simulink model "soc_dvbs2_fpga"  (R2025b)
settings: Solver=FixedStepDiscrete  StartTime=0.0  StopTime=0  RelTol=1e-3
InitFcn:
  | soc_dvbs2_init;
values from neighbouring files (symbols this model uses):
  Rsym = 4e6    (= 4000000)    [soc_dvbs2_init.m]
  soc_dvbs2_txPacketBits = [1 1 0 1 0 1 1 1 0 1 1 1 ... (2972 elements, 2972x1)]    [soc_dvbs2_txPacketBits.mat]
  syncWord = (dec2bin(hex2dec('AC')) - '0').'    [soc_dvbs2_init.m]
  txDataOut = txobj(frameBits(:))    [soc_dvbs2_init.m]
  txFiltCoeff = txobj.pTxFilterCoeff    [soc_dvbs2_init.m]
undefined symbols (not defined in the file or in its folder): Add, coefficientsLog, coefficientsSqrt1, coefficientsSqrt2, dataBits, designMultirateFIR, noisePow, NumBits1, NumBits2, seedsURNG1, seedsURNG2, Shift, Slope1, Slope2, soc_dvbs2_designFIRFilter, txDataOutS1, txDataOutS10, txDataOutS12, txDataOutS13, txDataOutS14, txDataOutS15, txDataOutS16, txDataOutS18, txDataOutS19, txDataOutS2, txDataOutS20, txDataOutS21, txDataOutS22, txDataOutS24, txDataOutS25, txDataOutS26, txDataOutS27, txDataOutS3, txDataOutS4, txDataOutS5, txDataOutS6, txDataOutS7, txDataOutS8, txDataOutS9
libraries: simulink x214, hdlsllib x211, dspsigops x22, dsphdlfiltering2 x8, dsphdlsigops2 x5, commseqgen3 x5, dsphdlmathfun2 x3, hwlogicconnlib x2, whdledac x2, commhdlcrc x2, whdlutilities x1, whdlmod x1
(part 12 of 12)

== matlab function soc_dvbs2_fpga/DVBS2/DVBS2 TxRx/DVB-S2 HDL Receiver/Demod Deinterleave and FECDecode/DVBS2 HDL Deinterleaver/RAM Address Generator/Read Offset Address/Read Offset Address Signals Generator ==
  data: maxR input; chkwrAddrEnd input; maxC input; modcodIs12 input; wrAddr input; curCorROut output; maxRorCOut output; curRorCOut output; modcodIs12Out output; startOut output; endOut output; wrEnb input; readValid output; isInterleave parameter
function [curCorROut,maxRorCOut,curRorCOut,modcodIs12Out,startOut,endOut,readValid] = readAddrCtrl(maxR,chkwrAddrEnd,maxC,modcodIs12,wrAddr,wrEnb,isInterleave)
%#codegen

    persistent rdEnb rdEnbOld startOutReg;
    persistent curR curC vMaxR vMaxC wrIdx rdIdx;
    persistent framCnt vModCodIs12;
    persistent curCorROutReg maxRorCOutReg curRorCOutReg modcodIs12OutReg;

    if isempty(rdEnb)
        rdEnb           = false;
%         rdEnbPrev       = false;
        rdEnbOld        = false;
        curR            = cast(0,'like',maxR);
        curC            = cast(0,'like',maxC);
        wrIdx           = fi(0,0,3,0,hdlfimath);
        rdIdx           = fi(0,0,3,0,hdlfimath);
        vMaxR           = cast(zeros(8,1),'like',maxR);
        vMaxC           = cast(zeros(8,1),'like',maxC);
        vModCodIs12     = false(8,1);
        startOutReg     = false;
        framCnt         = fi(0,0,3,0,hdlfimath);
        
        % XorY => Store X for Interleaver and Y for Deinterleaver
        if isInterleave        
            curCorROutReg   = curC;
            maxRorCOutReg   = vMaxR(1);
            curRorCOutReg   = curR;
        else
            curCorROutReg   = curR;
            maxRorCOutReg   = vMaxC(1);
            curRorCOutReg   = curC;
        end
        
        modcodIs12OutReg = vModCodIs12(1);
    end
    
    curCorROut   = curCorROutReg;
    maxRorCOut   = maxRorCOutReg;
    curRorCOut   = curRorCOutReg;
    modcodIs12Out = modcodIs12OutReg;
    readValid = rdEnbOld;
    startOut  = startOutReg; 
    
    endOut = false;
    if rdEnbOld
        if (isInterleave && (curC == (vMaxC(rdIdx+1)-1))) || (~isInterleave && (curR == (vMaxR(rdIdx+1)-1)))
            if isInterleave
                curC(:) = 0;
            else
                curR(:) = 0;
            end 
            if (~isInterleave && (curC == (vMaxC(rdIdx+1)-1))) || (isInterleave && (curR == (vMaxR(rdIdx+1)-1)))
                if ~isInterleave
                    curC(:) = 0;
                else
                    curR(:) = 0;
                end
                framCnt(:) = framCnt - 1;
                if framCnt == 0
                    rdEnb(:) = false;
                end
                endOut = true;
                if rdIdx == 7
                    rdIdx(:) = 0;
                else
                    rdIdx(:) = rdIdx + 1;
                end
            else
                if isInterleave
                    curR(:) = curR + 1;
                else
                    curC(:) = curC + 1;
                end
            end
        else
            if isInterleave
                curC(:) = curC + 1;
            else
                curR(:) = curR + 1;
            end
        end
    end
    
    if vModCodIs12(rdIdx+1) && curC == 0
        curCAdj = cast(2,'like',curC);
    elseif vModCodIs12(rdIdx+1) && curC == 2
        curCAdj = cast(0,'like',curC);
    else
        curCAdj = curC;
    end
    
    
    if isInterleave
        curCorROutReg    = curCAdj;
        maxRorCOutReg    = vMaxR(rdIdx+1);
        curRorCOutReg    = curR;
    else
        curCorROutReg    = curR;
        maxRorCOutReg    = vMaxC(rdIdx+1);
        curRorCOutReg    = curCAdj;
    end
    
    modcodIs12OutReg = vModCodIs12(rdIdx+1);

    startOutReg = rdEnb && (curR==0) && (curC==0);
    rdEnbOld = rdEnb;
%     rdEnbPrev = wrEnb && (wrAddr == chkwrAddrEnd);
    
    if wrEnb && (wrAddr == chkwrAddrEnd)
        framCnt(:) = framCnt + 1;
        rdEnb(:) = true;
        vModCodIs12(wrIdx+1) = modcodIs12;
        vMaxR(wrIdx+1) = maxR;
        vMaxC(wrIdx+1) = maxC;
        if wrIdx == 7
            wrIdx(:) = 0;
        else
            wrIdx(:) = wrIdx + 1;
        end
    end
    
end

== matlab function soc_dvbs2_fpga/DVBS2/DVBS2 TxRx/Channel/AWGN Generator/Unit Variance Gaussian Noise/logImplementation/log/RangeReduction/leadingZeroDetector ==
  data: x input; exp_e output
function exp_e=leadingZeroDetector(x)
temp = 0;
flag=1.0e+14 *[0.000000000000020
   0.000000000000040
   0.000000000000080
   0.000000000000160
   0.000000000000320
   0.000000000000640
   0.000000000001280
   0.000000000002560
   0.000000000005120
   0.000000000010240
   0.000000000020480
   0.000000000040960
   0.000000000081920
   0.000000000163840
   0.000000000327680
   0.000000000655360
   0.000000001310720
   0.000000002621440
   0.000000005242880
   0.000000010485760
   0.000000020971520
   0.000000041943040
   0.000000083886080
   0.000000167772160
   0.000000335544320
   0.000000671088640
   0.000001342177280
   0.000002684354560
   0.000005368709120
   0.000010737418240
   0.000021474836480
   0.000042949672960
   0.000085899345920
   0.000171798691840
   0.000343597383680
   0.000687194767360
   0.001374389534720
   0.002748779069440
   0.005497558138880
   0.010995116277760
   0.021990232555520
   0.043980465111040
   0.087960930222080
   0.175921860444160
   0.351843720888320
   0.703687441776640
   1.407374883553280
   2.814749767106560];

% else
%     while( )
%         temp = temp+1;
%         flag()=flag()*2;
%     end
% end
% 
% end
if(x == 0)
     temp = 49;
elseif (x*flag(1)>1)
        temp=1;
elseif (x*flag(2)>1)
        temp=2;
elseif (x*flag(3)>1)
        temp=3;
elseif (x*flag(4)>1)
        temp=4;
elseif (x*flag(5)>1)
        temp=5;
elseif (x*flag(6)>1)
        temp=6;
elseif (x*flag(7)>1)
        temp=7;
elseif (x*flag(8)>1)
        temp=8;
elseif (x*flag(9)>1)
        temp=9;
elseif (x*flag(10)>1)
        temp=10;
elseif (x*flag(11)>1)
        temp=11;
elseif (x*flag(12)>1)
        temp=12;
elseif (x*flag(13)>1)
        temp=13;
elseif (x*flag(14)>1)
        temp=14;
elseif (x*flag(15)>1)
        temp=15;
elseif (x*flag(16)>1)
        temp=16;
elseif (x*flag(17)>1)
        temp=17;
elseif (x*flag(18)>1)
        temp=18;
elseif (x*flag(19)>1)
        temp=19;
elseif (x*flag(20)>1)
        temp=20;
elseif (x*flag(21)>1)
        temp=21;
elseif (x*flag(22)>1)
        temp=22;
elseif (x*flag(23)>1)
        temp=23;
elseif (x*flag(24)>1)
        temp=24;
elseif (x*flag(25)>1)
        temp=25;
elseif (x*flag(26)>1)
        temp=26;
elseif (x*flag(27)>1)
        temp=27;
elseif (x*flag(28)>1)
        temp=28;
elseif (x*flag(29)>1)
        temp=29;
elseif (x*flag(30)>1)
        temp=30;
elseif (x*flag(31)>1)
        temp=31;
elseif (x*flag(32)>1)
        temp=32;
elseif (x*flag(33)>1)
        temp=33;
elseif (x*flag(34)>1)
        temp=34;
elseif (x*flag(35)>1)
        temp=35;
elseif (x*flag(36)>1)
        temp=36;
elseif (x*flag(37)>1)
        temp=37;
elseif (x*flag(38)>1)
        temp=8;
elseif (x*flag(39)>1)
        temp=39;
elseif (x*flag(40)>1)
        temp=40;
elseif (x*flag(41)>1)
        temp=41;
elseif (x*flag(42)>1)
        temp=42;
elseif (x*flag(43)>1)
        temp=43;
elseif (x*flag(44)>1)
        temp=44;
elseif (x*flag(45)>1)
        temp=45;
elseif (x*flag(46)>1)
        temp=46;
elseif (x*flag(47)>1)
        temp=47; 
elseif (x*flag(48)>1)
        temp=48; 
end        
exp_e=uint8(temp);

== matlab function soc_dvbs2_fpga/DVBS2/DVBS2 TxRx/DVB-S2 HDL Receiver/Synchronizer and PL Header Decoder/Source Encoding/MATLAB Function ==
  data: In input; out output; isdummy output
function [out,isdummy] = fcn(In)


if (In == 0)
    out = fi(0,0,2,0);
    isdummy = true;    
elseif (In <= 11)
    out = fi(0,0,2,0);
    isdummy = false;
elseif (In <= 17)
    out = fi(1,0,2,0);
    isdummy = false;
elseif (In <= 23)
    out = fi(2,0,2,0);
    isdummy = false;
elseif (In <= 28)
    out = fi(3,0,2,0);
    isdummy = false;
else
    out = fi(0,0,2,0);
    isdummy = true;
end

== matlab function soc_dvbs2_fpga/DVBS2/DVBS2 TxRx/DVB-S2 HDL Receiver/Synchronizer and PL Header Decoder/Time Frequency and Coarse Phase Synchronizer/Time and Coarse Frequency Synchronizer/Frame Synchronizer/Pilot and Sync Pulse Indicator/ThresholdLimiter ==
  settings: fimath=hdlfimath
  data: x input; y output
function y = applyLowerLimit(x)
    % Apply a lower limit to the threshold.
    %#codegen
    
    % Threshold is computed by summing across 63 samples.
    % Set lower limit to be equivalent of all 63 samples
    % having their LSB set to 1 and all others set to 0. 
    lowerLimit = cast(64 * 2^-x.FractionLength, 'like', x); % use 64 for HDL
    
    if x < lowerLimit
        y = lowerLimit;
    else
        y = x;
    end
end

== matlab function soc_dvbs2_fpga/DVBS2/DVBS2 TxRx/DVB-S2 HDL Receiver/Synchronizer and PL Header Decoder/Time Frequency and Coarse Phase Synchronizer/Time and Coarse Frequency Synchronizer/Symbol Synchronizer/Interpolation Control ==
  data: mu output; Delta input; Underflow output
function [mu,Underflow] = Interpolation_ctrl(Delta)
% Implementation of modulo-1 counter for interpolation control listed in
% Figure 8.4.19 of "Digital Communications - A Discrete-Time Approach"
% by Michael Rice. See design details in Chapter 8.4.3 of the same book.
% 
% Input:
%   Delta - Loop filter output. If loop is in lock, delta would be small
% Output:
%   Underflow - Indicator of counter underflow. This is the strobe signal
%               for downstream processing
%   mu - Difference between actual sampling instant and the optimal instant,
%        between zero and one
%#codegen

% countReg - Counter value delayed by 1 sample
% muReg - The estimated timing error normalized by half QPSK symbols

   mask = fi(1-2^(-10),1,11,10);
   
   persistent countReg underflowReg muReg;
   if isempty(countReg)
       countReg  = fi(0,1,11,10);
       muReg = fi(0,1,11,10);
       underflowReg = false;
   end
   
   
   Underflow = underflowReg;
   mu = muReg;   
   
   
   counter = bitand(mask,countReg)-Delta-fi(0.25,1,11,10); % decrementing counter
   
   % if countReg is a nonnegative number,
   % then mod(countReg,1) equals the fractional part of countReg
   if counter < 0
       underflowReg = true;
       muReg = bitshift(bitand(mask,countReg),2);
       countReg = fi(counter+1,1,11,10);% create underflow to counter
   else
       underflowReg = false;
       countReg = fi(counter,1,11,10);
   end
   


end

== matlab function soc_dvbs2_fpga/DVBS2/DVBS2 TxRx/DVB-S2 HDL Receiver/Synchronizer and PL Header Decoder/Time Frequency and Coarse Phase Synchronizer/Time and Coarse Frequency Synchronizer/Symbol Synchronizer/Rate Handle/FIFO/MATLAB Function ==
  data: wr input; full output; rd input; empty output
function [full,empty] = fcn(wr,rd)
%#codegen
     
    WL = nextpow2(1024-1);
    maxCountVal = fi(2^(WL+1) - 1,0,WL+1,0);
    persistent count;
    if isempty(count)
        count = fi(0,0,WL+1,0,hdlfimath);
    end

   

    if wr
        if count == maxCountVal
            count(:) = 0;
        else
            count(:) = count + 1;
        end
    end
    if rd
        if count == 0
            count(:) = maxCountVal;
        else
            count(:) = count - 1;
        end
    end


    empty = (count == 0);
    full = (count > 2^WL-1);
    % ncount = count;

end
